simulink model "loopback_delay_estimation"  (R2019b)
settings: Solver=VariableStepAuto  StartTime=0.0  StopTime=18000  RelTol=1e-3
InitFcn:
  | initScript
values from neighbouring files (symbols this model uses):
  bool_ref = (tx_input_ampl_diff<0)    [initScript.m]
  cst = round(scale*cst)    [initScript.m]
  len2 = (len1+d)*L    (= 200)    [initScript.m]
  scale = 30000    [find_corr_threshold.m]    (also in initScript.m = 25000; run_loopback_tests.m = 28000)
  sync_seq_im = int16([cst_im zc_im.' zeros(1, 6000)])    [initScript.m]
  sync_seq_re = int16([cst_re zc_re.' zeros(1, 6000)])    [initScript.m]
  zc_re = round(scale*zc_re/max_val_re)    [initScript.m]
undefined symbols (not defined in the file or in its folder): j
libraries: hdlsllib x11, simulink x6, dsphdlmathfun x2, commsource2 x1, dspsigops x1, commrflib2 x1
settings Model: SimulationMode=accelerator  Creator=spagadar  LastModifiedBy=spagadar
settings OptimizationCC: BlockReduction=off  ConditionallyExecuteInputs=off  DefaultParameterBehavior=Inlined
settings DebuggingCC: AlgebraicLoopMsg=error
settings HardwareCC: ProdBitPerPointer=32  ProdBitPerSizeT=32  ProdBitPerPtrDiffT=32  ProdLargestAtomicFloat=None  ProdIntDivRoundTo=Undefined  ProdEndianess=Unspecified  ProdWordSize=32  ProdHWDeviceType=ASIC/FPGA->ASIC/FPGA  TargetBitPerPointer=64  TargetBitPerSizeT=64  TargetBitPerPtrDiffT=64  TargetLongLongMode=on  TargetIntDivRoundTo=Zero  TargetEndianess=LittleEndian  TargetWordSize=64  TargetHWDeviceType=Custom Processor->MATLAB Host Computer  ProdEqTarget=off

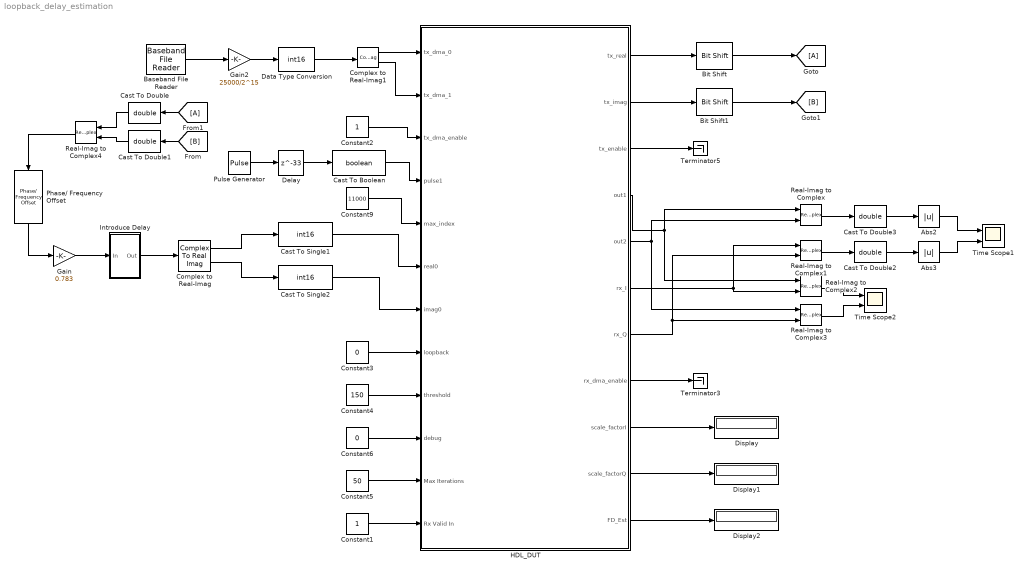
== system loopback_delay_estimation ==
  Abs2 : Abs
  Abs3 : Abs
  Baseband File Reader : commsource2/Baseband File Reader  Filename=zc_out_data_fd.bb  InheritSampleTimeFromFile=on  SampleTime=1  SamplesPerFrame=1  CyclicRepetition=off  FileEndOutputPort=off  SimulateUsing=Code generation
      settings: SourceProductName=Communications Toolbox  SourceProductBaseCode=CM
  Bit Shift : hdlsllib/Logic and Bit Operations/Bit Shift  mode=Shift Right Arithmetic  N=4
      settings: SourceProductName=Simulink
  Bit Shift1 : hdlsllib/Logic and Bit Operations/Bit Shift  mode=Shift Right Arithmetic  N=4
      settings: SourceProductName=Simulink
  Cast To Boolean : DataTypeConversion  OutDataTypeStr=boolean
  Cast To Double{,1..3} (4 alike) : DataTypeConversion  OutDataTypeStr=double
  Cast To Single1 : DataTypeConversion  OutDataTypeStr=int16
  Cast To Single2 : DataTypeConversion  OutDataTypeStr=int16
  Complex to Real-Imag : ComplexToRealImag
  Complex to Real-Imag1 : ComplexToRealImag
  Constant1 : Constant  OutDataTypeStr=boolean  SampleTime=-1
  Constant2 : Constant  OutDataTypeStr=boolean  SampleTime=-1
  Constant3 : Constant  Value=0  OutDataTypeStr=boolean  SampleTime=-1
  Constant4 : Constant  Value=150  OutDataTypeStr=uint16  SampleTime=-1
  Constant5 : Constant  Value=50  OutDataTypeStr=uint16  SampleTime=-1
  Constant6 : Constant  Value=0  OutDataTypeStr=uint16  SampleTime=-1
  Constant9 : Constant  Value=11000  OutDataTypeStr=uint32  SampleTime=-1
  Data Type Conversion : DataTypeConversion  OutDataTypeStr=int16
  Delay : Delay  DelayLength=33
  Display : Display
  Display1 : Display
  Display2 : Display
  Gain : Gain  Gain=0.783
  Gain2 : Gain  Gain=25000/2^15
  HDL_DUT : Subsystem  TreatAsAtomicUnit=on
  Introduce Delay : Subsystem  mask{fd=10, id=146}
      mask prompts: fd "Fractional Delay"; id "Integer Delay"
      mask DialogControl DescTextVar Prompt: Introduce Delay
  Phase/ Frequency Offset : commrflib2/Phase// Frequency Offset  phaseOffset=0  freqPort=off  freqOffset=0
      settings: SourceProductName=Communications Toolbox
  Pulse Generator : DiscretePulseGenerator  Period=16000
  Real-Imag to Complex{,1..4} (5 alike) : RealImagToComplex
  Terminator3 : Terminator
  Terminator5 : Terminator
  Time Scope1 : Scope  NumInputPorts=2
  Time Scope2 : Scope  NumInputPorts=2
  wires:
  [A] -> Cast To Double/1
  [B] -> Cast To Double1/1
  Constant9/1 -> HDL_DUT/5(max_index)
  Complex to Real-Imag/1 -> Cast To Single1/1
  Data Type Conversion/1 -> Complex to Real-Imag1/1
  Constant6/1 -> HDL_DUT/10(debug)
  Complex to Real-Imag1/2 -> HDL_DUT/2(tx_dma_1)
  Cast To Double1/1 -> Real-Imag to Complex4/2
  Cast To Double/1 -> Real-Imag to Complex4/1
  Complex to Real-Imag1/1 -> HDL_DUT/1(tx_dma_0)
  Constant2/1 -> HDL_DUT/3(tx_dma_enable)
  HDL_DUT/1(tx_real) -> Bit Shift/1
  HDL_DUT/2(tx_imag) -> Bit Shift1/1
  Complex to Real-Imag/2 -> Cast To Single2/1
  Constant3/1 -> HDL_DUT/8(loopback)
  Phase/ Frequency Offset/1 -> Gain/1
  Constant4/1 -> HDL_DUT/9(threshold)
  HDL_DUT/8(rx_dma_enable) -> Terminator3/1
  Baseband File Reader/1 -> Gain2/1
  HDL_DUT/3("tx_enable ") -> Terminator5/1
  HDL_DUT/6(rx_I) -> Real-Imag to Complex2/2, Real-Imag to Complex1/1
  HDL_DUT/7(rx_Q) -> Real-Imag to Complex3/2, Real-Imag to Complex1/2
  HDL_DUT/4(out1) -> Real-Imag to Complex2/1, Real-Imag to Complex/1
  HDL_DUT/5(out2) -> Real-Imag to Complex3/1, Real-Imag to Complex/2
  Constant5/1 -> HDL_DUT/11(Max Iterations)
  Abs2/1 -> Time Scope1/1
  Abs3/1 -> Time Scope1/2
  Real-Imag to Complex/1 -> Cast To Double3/1
  Real-Imag to Complex1/1 -> Cast To Double2/1
  Cast To Double2/1 -> Abs3/1
  Cast To Double3/1 -> Abs2/1
  Cast To Single1/1 -> HDL_DUT/6(real0)
  Cast To Single2/1 -> HDL_DUT/7(imag0)
  HDL_DUT/9(scale_factorI) -> Display/1
  Constant1/1 -> HDL_DUT/12(Rx Valid In)
  Real-Imag to Complex2/1 -> Time Scope2/1
  Real-Imag to Complex3/1 -> Time Scope2/2
  HDL_DUT/10(scale_factorQ) -> Display1/1
  Gain2/1 -> Data Type Conversion/1
  HDL_DUT/11(FD_Est) -> Display2/1
  Pulse Generator/1 -> Delay/1
  Cast To Boolean/1 -> HDL_DUT/4(pulse1)
  Delay/1 -> Cast To Boolean/1
  Real-Imag to Complex4/1 -> Phase/ Frequency Offset/1
  Bit Shift/1 -> [A]
  Bit Shift1/1 -> [B]
  Introduce Delay/1(Out) -> Complex to Real-Imag/1
  Gain/1 -> Introduce Delay/1(In)

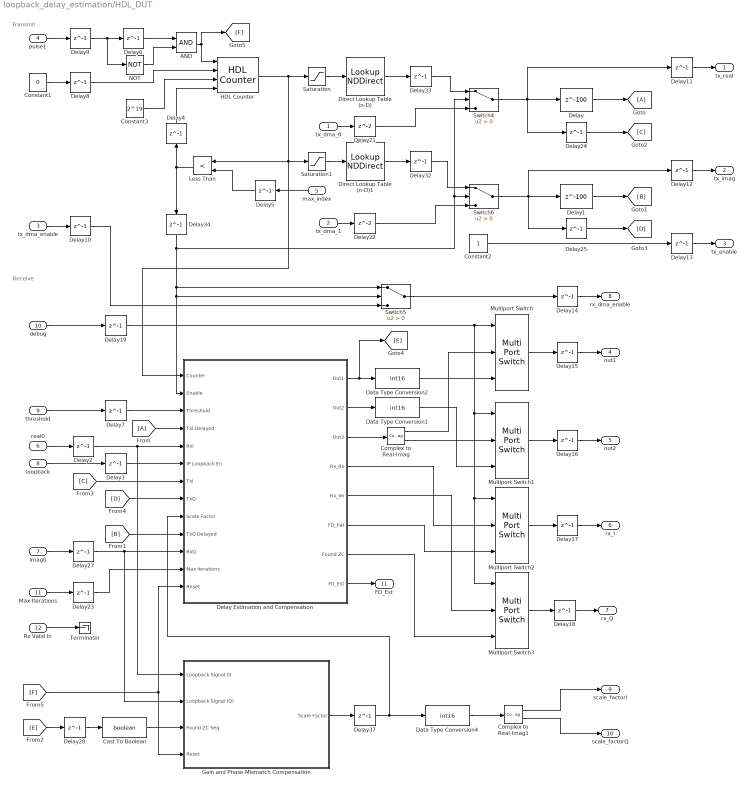
== system loopback_delay_estimation/HDL_DUT ==
  note: Receive
  note: Transmit
  tx_dma_0 : Inport
  tx_dma_1 : Inport  Port=2
  tx_dma_enable : Inport  Port=3
  pulse1 : Inport  Port=4
  max_index : Inport  Port=5  OutDataTypeStr=uint32
  real0 : Inport  Port=6
  imag0 : Inport  Port=7
  loopback : Inport  Port=8  OutDataTypeStr=boolean
  threshold : Inport  Port=9  OutDataTypeStr=uint16
  debug : Inport  Port=10
  Max Iterations : Inport  Port=11  OutDataTypeStr=uint16
  Rx Valid In : Inport  Port=12
  AND : Logic  AllPortsSameDT=off  OutDataTypeStr=boolean
  Cast To Boolean : DataTypeConversion  OutDataTypeStr=boolean
  Complex to Real-Imag : ComplexToRealImag
  Complex to Real-Imag1 : ComplexToRealImag
  Constant1 : Constant  Value=0  OutDataTypeStr=boolean  SampleTime=-1
  Constant2 : Constant  OutDataTypeStr=boolean  SampleTime=-1
  Constant3 : Constant  Value=2^19  OutDataTypeStr=uint32  SampleTime=-1
  Data Type Conversion1 : DataTypeConversion  OutDataTypeStr=int16
  Data Type Conversion2 : DataTypeConversion  OutDataTypeStr=int16
  Data Type Conversion4 : DataTypeConversion  OutDataTypeStr=int16
  Delay : Delay  DelayLength=100  InitialCondition=0  UseCircularBuffer=on
  Delay Estimation and Compensation : Subsystem
  Delay1 : Delay  DelayLength=100  InitialCondition=0  UseCircularBuffer=on
  Delay{2..7,9..19,23..25,27..28,32..34,37} (26 alike) : Delay  DelayLength=1
  Delay21 : Delay
  Delay22 : Delay
  Delay8 : Delay  DelayLength=1  InitialCondition=1
  Direct Lookup Table (n-D) : LookupNDDirect  NumberOfTableDimensions=1  Table=sync_seq_re  DiagnosticForOutOfRangeInput=Error  TableDataTypeStr=int16
  Direct Lookup Table (n-D)1 : LookupNDDirect  NumberOfTableDimensions=1  Table=sync_seq_im  DiagnosticForOutOfRangeInput=Error  TableDataTypeStr=int16
  Gain and Phase Mismatch Compensation : Subsystem
  HDL Counter : hdlsllib/Sources/HDL Counter  CountType=Count limited  CountInit=0  CountStep=1  CountMax=2^20  CountFromType=Initial value  CountFrom=0  CountResetPort=on  CountLoadPort=on  CountEnbPort=on  CountDirPort=off  CountDataType=Unsigned  CountWordLen=32  CountFracLen=0  CountSampTime=1
      settings: SourceProductBaseCode=HD
  Less Than : RelationalOperator  Operator=<  OutDataTypeStr=boolean  RndMeth=Simplest
  Multiport Switch{,1..3} (4 alike) : MultiPortSwitch  DataPortOrder=Zero-based contiguous  Inputs=2  zeroidx=on  OutDataTypeStr=int16
  NOT : Logic  Operator=NOT  IconShape=distinctive  AllPortsSameDT=off  OutDataTypeStr=boolean
  Saturation : Saturate  UpperLimit=999  LowerLimit=0
  Saturation1 : Saturate  UpperLimit=999  LowerLimit=0
  Switch4 : Switch  Criteria=u2 > Threshold
  Switch5 : Switch  Criteria=u2 > Threshold
  Switch6 : Switch  Criteria=u2 > Threshold
  Terminator : Terminator
  tx_real : Outport  VectorParamsAs1DForOutWhenUnconnected=off
  tx_imag : Outport  Port=2  VectorParamsAs1DForOutWhenUnconnected=off
  "tx_enable " : Outport  Port=3  VectorParamsAs1DForOutWhenUnconnected=off
  out1 : Outport  Port=4  OutDataTypeStr=int16  VectorParamsAs1DForOutWhenUnconnected=off
  out2 : Outport  Port=5  VectorParamsAs1DForOutWhenUnconnected=off
  rx_I : Outport  Port=6  VectorParamsAs1DForOutWhenUnconnected=off
  rx_Q : Outport  Port=7  VectorParamsAs1DForOutWhenUnconnected=off
  rx_dma_enable : Outport  Port=8  VectorParamsAs1DForOutWhenUnconnected=off
  scale_factorI : Outport  Port=9  VectorParamsAs1DForOutWhenUnconnected=off
  scale_factorQ : Outport  Port=10  VectorParamsAs1DForOutWhenUnconnected=off
  FD_Est : Outport  Port=11  VectorParamsAs1DForOutWhenUnconnected=off
  wires:
  Direct Lookup Table (n-D)/1 -> Delay33/1
  tx_dma_0/1 -> Delay21/1
  Constant2/1 -> Delay13/1
  loopback/1 -> Delay3/1
  Delay/1 -> [A]
  Delay1/1 -> [B]
  Switch5/1 -> Delay14/1
  tx_dma_enable/1 -> Delay10/1
  Switch4/1 -> Delay11/1, Delay24/1, Delay/1
  Direct Lookup Table (n-D)1/1 -> Delay32/1
  Switch6/1 -> Delay12/1, Delay1/1, Delay25/1
  tx_dma_1/1 -> Delay22/1
  Saturation/1 -> Direct Lookup Table (n-D)/1
  pulse1/1 -> Delay9/1
  Delay6/1 -> AND/1
  NOT/1 -> AND/2
  AND/1 -> [F], HDL Counter/1
  Delay9/1 -> NOT/1, Delay6/1
  Delay10/1 -> Switch5/3
  Delay11/1 -> tx_real/1
  Delay12/1 -> tx_imag/1
  Delay13/1 -> "tx_enable "/1
  Delay14/1 -> rx_dma_enable/1
  Delay15/1 -> out1/1
  Delay16/1 -> out2/1
  Delay17/1 -> rx_I/1
  Delay18/1 -> rx_Q/1
  max_index/1 -> Delay5/1
  Delay21/1 -> Switch4/3
  Delay22/1 -> Switch6/3
  Less Than/1 -> Delay4/1, Delay34/1
  Delay24/1 -> [C]
  Delay25/1 -> [D]
  Delay32/1 -> Switch6/1
  Delay33/1 -> Switch4/1
  Delay4/1 -> HDL Counter/4
  Delay5/1 -> Less Than/2
  [E] -> Delay28/1
  Gain and Phase Mismatch Compensation/1("Scale Factor ") -> Delay37/1
  real0/1 -> Delay2/1
  imag0/1 -> Delay27/1
  Max Iterations/1 -> Delay23/1
  Multiport Switch/1 -> Delay15/1
  Multiport Switch1/1 -> Delay16/1
  Delay28/1 -> Cast To Boolean/1
  Delay Estimation and Compensation/3(Out3) -> Complex to Real-Imag/1
  Delay Estimation and Compensation/2(Out2) -> Data Type Conversion1/1
  Delay Estimation and Compensation/1(Out1) -> [E], Data Type Conversion2/1
  Delay23/1 -> Delay Estimation and Compensation/12(Max Iterations)
  Delay27/1 -> Delay Estimation and Compensation/11(RxQ), Gain and Phase Mismatch Compensation/2(Loopback Signal (Q))
  [B] -> Delay Estimation and Compensation/10(TxQ Delayed)
  Delay37/1 -> Data Type Conversion4/1, Delay Estimation and Compensation/9(Scale Factor)
  [D] -> Delay Estimation and Compensation/8(TxQ)
  [C] -> Delay Estimation and Compensation/7(TxI)
  Delay2/1 -> Delay Estimation and Compensation/5(RxI), Gain and Phase Mismatch Compensation/1(Loopback Signal (I))
  Delay3/1 -> Delay Estimation and Compensation/6(IP Loopback En)
  [A] -> Delay Estimation and Compensation/4(TxI Delayed)
  Delay7/1 -> Delay Estimation and Compensation/3(Threshold)
  Delay34/1 -> Delay Estimation and Compensation/2(Enable), Switch5/2, Switch5/1, Switch4/2, Switch6/2
  Data Type Conversion1/1 -> Multiport Switch1/3
  Data Type Conversion2/1 -> Multiport Switch/3
  HDL Counter/1 -> Saturation1/1, Delay Estimation and Compensation/1(Counter), Less Than/1, Saturation/1
  threshold/1 -> Delay7/1
  Delay19/1 -> Multiport Switch3/1, Multiport Switch2/1, Multiport Switch1/1, Multiport Switch/1
  debug/1 -> Delay19/1
  Multiport Switch3/1 -> Delay18/1
  Multiport Switch2/1 -> Delay17/1
  Delay Estimation and Compensation/4(Rx_Re) -> Multiport Switch2/2
  Delay Estimation and Compensation/5(Rx_Im) -> Multiport Switch3/2
  Cast To Boolean/1 -> Gain and Phase Mismatch Compensation/3(Found ZC Seq)
  Complex to Real-Imag/1 -> Multiport Switch/2
  Complex to Real-Imag/2 -> Multiport Switch1/2
  Rx Valid In/1 -> Terminator/1
  Saturation1/1 -> Direct Lookup Table (n-D)1/1
  Data Type Conversion4/1 -> Complex to Real-Imag1/1
  Complex to Real-Imag1/1 -> scale_factorI/1
  Complex to Real-Imag1/2 -> scale_factorQ/1
  Constant1/1 -> Delay8/1
  Delay8/1 -> HDL Counter/2
  Constant3/1 -> HDL Counter/3
  Delay Estimation and Compensation/8(FD_Est) -> FD_Est/1
  [F] -> Delay Estimation and Compensation/13(Reset), Gain and Phase Mismatch Compensation/4(Reset)
  Delay Estimation and Compensation/6(FD_hat) -> Multiport Switch2/3
  Delay Estimation and Compensation/7(Found ZC) -> Multiport Switch3/3

== system loopback_delay_estimation/Introduce Delay ==
  In : Inport
  Constant8 : Constant  Value=fd/16
  Delay : Delay  DelayLength=id  InitialCondition=0  UseCircularBuffer=on
  Variable Fractional Delay : dspsigops/Variable Fractional Delay  mode=OBSOLETE  modeActive=Linear  L=4  FarrowL=4  R=10  alpha=1  dmax=100  InputProcessing=Columns as channels (frame based)  ic=0  noDFT=off  fallbackFIR=Clip to the minimum value necessary for centered kernel  fallbackFarrow=Clip to the minimum value necessary for centered kernel  roundingMode=Zero  overflowMode=off
      settings: SourceProductName=DSP System Toolbox  SourceProductBaseCode=DS
  Out : Outport  VectorParamsAs1DForOutWhenUnconnected=off
  wires:
  Constant8/1 -> Variable Fractional Delay/2
  In/1 -> Delay/1
  Delay/1 -> Variable Fractional Delay/1
  Variable Fractional Delay/1 -> Out/1

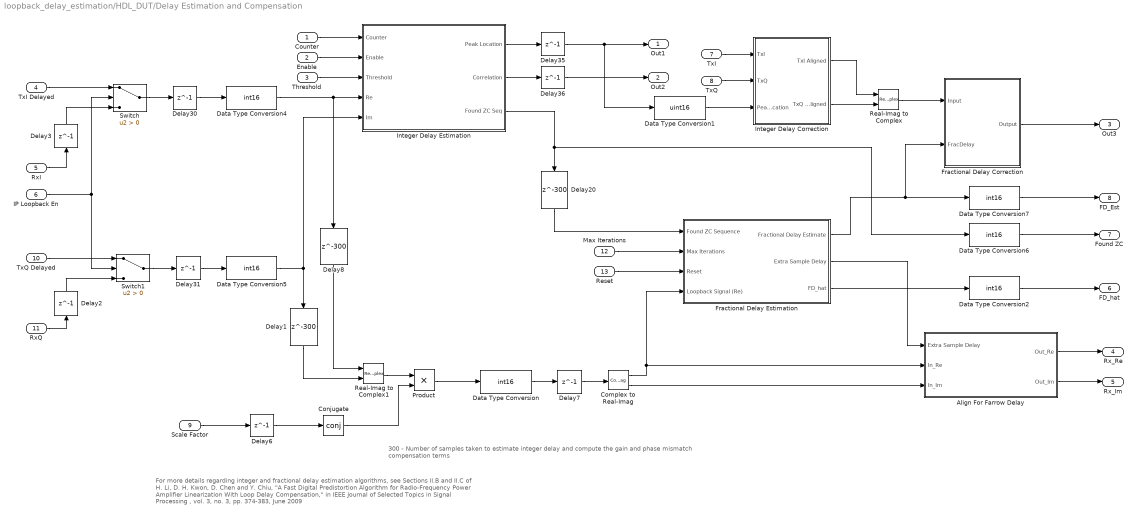
== system loopback_delay_estimation/HDL_DUT/Delay Estimation and Compensation ==
  note: For more details regarding integer and fractional delay estimation algorithms, see Sections II.B and II.C of
      | H. Li, D. H. Kwon, D. Chen and Y. Chiu, "A Fast Digital Predistortion Algorithm for Radio-Frequency Power Amplifier Linearization With Loop Delay Compensation," in IEEE Journal of Selected Topics in Signal Processing , vol. 3, no. 3, pp. 374-383, June 2009
  note: 300 - Number of samples taken to estimate integer delay and compute the gain and phase mismatch compensation terms
  Counter : Inport
  Enable : Inport  Port=2
  Threshold : Inport  Port=3
  TxI Delayed : Inport  Port=4
  RxI : Inport  Port=5
  IP Loopback En : Inport  Port=6
  TxI : Inport  Port=7
  TxQ : Inport  Port=8
  Scale Factor : Inport  Port=9
  TxQ Delayed : Inport  Port=10
  RxQ : Inport  Port=11
  Max Iterations : Inport  Port=12  OutDataTypeStr=uint16
  Reset : Inport  Port=13
  Align For Farrow Delay : Subsystem
  Complex to Real-Imag : ComplexToRealImag
  Conjugate : Math  Operator=conj  RndMeth=Zero  SaturateOnIntegerOverflow=on
  Data Type Conversion{,2,4..7} (6 alike) : DataTypeConversion  OutDataTypeStr=int16
  Data Type Conversion1 : DataTypeConversion  OutDataTypeStr=uint16
  Delay1 : Delay  DelayLength=300  InitialCondition=0  UseCircularBuffer=on
  Delay{2..3,6..7,30..31,35..36} (8 alike) : Delay  DelayLength=1
  Delay20 : Delay  DelayLength=300  InitialCondition=0  UseCircularBuffer=on
  Delay8 : Delay  DelayLength=300  InitialCondition=0  UseCircularBuffer=on
  Fractional Delay Correction : Subsystem  Tag=FilterWizardSubSystem
      settings: ErrorFcn=dspFilterRealizedInBasicElemsAlgLoopErrFcnCallback
  Fractional Delay Estimation : Subsystem
  Integer Delay Correction : Subsystem
  Integer Delay Estimation : Subsystem
  Product : Product
  Real-Imag to Complex : RealImagToComplex
  Real-Imag to Complex1 : RealImagToComplex
  Switch : Switch  Criteria=u2 > Threshold
  Switch1 : Switch  Criteria=u2 > Threshold
  Out1 : Outport
  Out2 : Outport  Port=2
  Out3 : Outport  Port=3
  Rx_Re : Outport  Port=4
  Rx_Im : Outport  Port=5
  FD_hat : Outport  Port=6
  Found ZC : Outport  Port=7
  FD_Est : Outport  Port=8  VectorParamsAs1DForOutWhenUnconnected=off
  wires:
  TxI/1 -> Integer Delay Correction/1(TxI)
  Data Type Conversion4/1 -> Delay8/1, Integer Delay Estimation/4(Re)
  Max Iterations/1 -> Fractional Delay Estimation/2(Max Iterations)
  Delay31/1 -> Data Type Conversion5/1
  Delay30/1 -> Data Type Conversion4/1
  Counter/1 -> Integer Delay Estimation/1(Counter)
  Integer Delay Correction/2(TxQ Aligned) -> Real-Imag to Complex/2
  Integer Delay Correction/1(TxI Aligned) -> Real-Imag to Complex/1
  Fractional Delay Estimation/1(Fractional Delay Estimate) -> Data Type Conversion7/1, Fractional Delay Correction/2(FracDelay)
  Data Type Conversion5/1 -> Integer Delay Estimation/5(Im), Delay1/1
  Fractional Delay Correction/1(Output) -> Out3/1
  Threshold/1 -> Integer Delay Estimation/3(Threshold)
  Delay35/1 -> Data Type Conversion1/1, Out1/1
  Switch1/1 -> Delay31/1
  Integer Delay Estimation/2(Correlation) -> Delay36/1
  Enable/1 -> Integer Delay Estimation/2(Enable)
  Delay36/1 -> Out2/1
  Real-Imag to Complex/1 -> Fractional Delay Correction/1(Input)
  TxQ Delayed/1 -> Switch1/1
  RxI/1 -> Delay3/1
  Integer Delay Estimation/1(Peak Location) -> Delay35/1
  TxI Delayed/1 -> Switch/1
  IP Loopback En/1 -> Switch1/2, Switch/2
  RxQ/1 -> Delay2/1
  TxQ/1 -> Integer Delay Correction/2(TxQ)
  Switch/1 -> Delay30/1
  Delay20/1 -> Fractional Delay Estimation/1(Found ZC Sequence)
  Delay3/1 -> Switch/3
  Delay2/1 -> Switch1/3
  Delay8/1 -> Real-Imag to Complex1/1
  Scale Factor/1 -> Delay6/1
  Delay1/1 -> Real-Imag to Complex1/2
  Data Type Conversion1/1 -> Integer Delay Correction/3(Peak Location)
  Complex to Real-Imag/1 -> Align For Farrow Delay/2(In_Re), Fractional Delay Estimation/4(Loopback Signal (Re))
  Data Type Conversion/1 -> Delay7/1
  Delay6/1 -> Conjugate/1
  Product/1 -> Data Type Conversion/1
  Delay7/1 -> Complex to Real-Imag/1
  Data Type Conversion2/1 -> FD_hat/1
  Conjugate/1 -> Product/2
  Real-Imag to Complex1/1 -> Product/1
  Data Type Conversion6/1 -> Found ZC/1
  Integer Delay Estimation/3(Found ZC Seq) -> Data Type Conversion6/1, Delay20/1
  Fractional Delay Estimation/3(FD_hat) -> Data Type Conversion2/1
  Fractional Delay Estimation/2(Extra Sample Delay) -> Align For Farrow Delay/1(Extra Sample Delay)
  Complex to Real-Imag/2 -> Align For Farrow Delay/3(In_Im)
  Align For Farrow Delay/1(Out_Re) -> Rx_Re/1
  Align For Farrow Delay/2(Out_Im) -> Rx_Im/1
  Reset/1 -> Fractional Delay Estimation/3(Reset)
  Data Type Conversion7/1 -> FD_Est/1

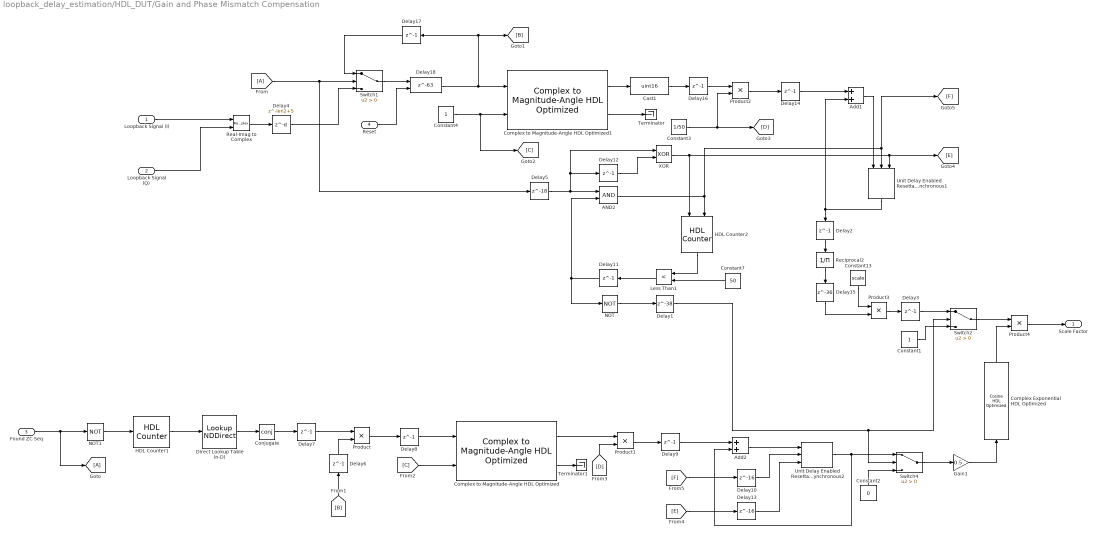
== system loopback_delay_estimation/HDL_DUT/Gain and Phase Mismatch Compensation ==
  Loopback Signal (I) : Inport
  Loopback Signal (Q) : Inport  Port=2
  Found ZC Seq : Inport  Port=3
  Reset : Inport  Port=4
  AND2 : Logic  AllPortsSameDT=off  OutDataTypeStr=boolean
  Add1 : Sum  OutDataTypeStr=uint32
  Add2 : Sum  OutDataTypeStr=fixdt(0,16,13)
  Cast1 : DataTypeConversion  OutDataTypeStr=uint16
  Complex Exponential HDL Optimized : hdlsllib/Lookup Tables/Cosine HDL Optimized  OutputFormula=exp(j*2*pi*u)  NumDataPoints=512  TableDataTypeStr=fixdt(0,16,15)  SimulateLUTROMDelay=off
      settings: SourceProductName=Simulink  SourceProductBaseCode=SL
  Complex to Magnitude-Angle HDL Optimized : dsphdlmathfun/Complex to Magnitude-Angle HDL Optimized  NumIterationsSource=Auto  NumIterations=10  OutputFormat=Angle  AngleFormat=Normalized  ScaleOutput=off  SimulateUsing=Code generation
      settings: SourceProductName=DSP System Toolbox  SourceProductBaseCode=DS
  Complex to Magnitude-Angle HDL Optimized1 : dsphdlmathfun/Complex to Magnitude-Angle HDL Optimized  NumIterationsSource=Auto  NumIterations=10  OutputFormat=Magnitude  AngleFormat=Radians  ScaleOutput=on  SimulateUsing=Code generation
      settings: SourceProductName=DSP System Toolbox  SourceProductBaseCode=DS
  Conjugate : Math  Operator=conj  RndMeth=Zero  SaturateOnIntegerOverflow=on
  Constant1 : Constant  OutDataTypeStr=uint16  SampleTime=-1
  Constant13 : Constant  Value=scale  OutDataTypeStr=uint16  SampleTime=-1
  Constant2 : Constant  Value=0  OutDataTypeStr=uint16  SampleTime=-1
  Constant3 : Constant  Value=1/50  OutDataTypeStr=fixdt(1,16,16)  SampleTime=-1
  Constant4 : Constant  OutDataTypeStr=boolean  SampleTime=-1
  Constant7 : Constant  Value=50  OutDataTypeStr=uint8  SampleTime=-1
  Delay1 : Delay  DelayLength=38
  Delay10 : Delay  DelayLength=16
  Delay{2..3,6..9,11..12,14,16..17} (11 alike) : Delay  DelayLength=1
  Delay13 : Delay  DelayLength=16
  Delay15 : Delay  DelayLength=36
  Delay18 : Delay  DelayLength=63  ExternalReset=Level
      settings: InputPortMap=u0,r5
  Delay4 : Delay  DelayLength=len2+5
  Delay5 : Delay  DelayLength=18
  Direct Lookup Table (n-D) : LookupNDDirect  NumberOfTableDimensions=1  Table=cst  DiagnosticForOutOfRangeInput=Error  TableDataTypeStr=int16
  Gain1 : Gain  Gain=0.5
  HDL Counter1 : hdlsllib/Sources/HDL Counter  CountType=Count limited  CountInit=0  CountStep=1  CountMax=63  CountFromType=Initial value  CountFrom=0  CountResetPort=on  CountLoadPort=off  CountEnbPort=off  CountDirPort=off  CountDataType=Unsigned  CountWordLen=8  CountFracLen=0  CountSampTime=1
      settings: SourceProductName=Simulink
  HDL Counter2 : hdlsllib/Sources/HDL Counter  CountType=Count limited  CountInit=0  CountStep=1  CountMax=60  CountFromType=Initial value  CountFrom=0  CountResetPort=on  CountLoadPort=off  CountEnbPort=on  CountDirPort=off  CountDataType=Unsigned  CountWordLen=8  CountFracLen=0  CountSampTime=1
      settings: SourceProductName=Simulink
  Less Than1 : RelationalOperator  Operator=<  OutDataTypeStr=boolean  RndMeth=Simplest
  NOT : Logic  Operator=NOT  AllPortsSameDT=off  OutDataTypeStr=boolean
  NOT1 : Logic  Operator=NOT  AllPortsSameDT=off  OutDataTypeStr=boolean
  Product{,1,3..4} (4 alike) : Product
  Product2 : Product  OutDataTypeStr=fixdt(0,16,7)
  Real-Imag to Complex : RealImagToComplex
  Reciprocal2 : Product  Inputs=/  SaturateOnIntegerOverflow=on  RndMeth=Zero
  Switch1 : Switch  Criteria=u2 > Threshold
  Switch2 : Switch  Criteria=u2 > Threshold  OutDataTypeStr=fixdt(0,16,7)
  Switch4 : Switch  Criteria=u2 > Threshold  OutDataTypeStr=fixdt(0,16,13)
  Terminator : Terminator
  Terminator1 : Terminator
  Unit Delay Enabled Resettable Synchronous1 : hdlsllib/Discrete/Unit Delay Enabled Resettable Synchronous  InitialCondition=0  SampleTime=-1
      settings: SourceProductName=Simulink  SourceProductBaseCode=SL
  Unit Delay Enabled Resettable Synchronous2 : hdlsllib/Discrete/Unit Delay Enabled Resettable Synchronous  InitialCondition=0  SampleTime=-1
      settings: SourceProductName=Simulink  SourceProductBaseCode=SL
  XOR : Logic  Operator=XOR  AllPortsSameDT=off  OutDataTypeStr=boolean
  "Scale Factor " : Outport
  wires:
  Loopback Signal (I)/1 -> Real-Imag to Complex/1
  Loopback Signal (Q)/1 -> Real-Imag to Complex/2
  Real-Imag to Complex/1 -> Delay4/1
  Reciprocal2/1 -> Delay15/1
  Less Than1/1 -> Delay11/1
  Unit Delay Enabled Resettable Synchronous1/1 -> Add1/2, Delay2/1
  HDL Counter2/1 -> Less Than1/1
  Constant7/1 -> Less Than1/2
  Constant3/1 -> [D], Product2/2
  Delay12/1 -> XOR/2
  Delay15/1 -> Product3/2
  Product2/1 -> Delay14/1
  Constant4/1 -> [C], Complex to Magnitude-Angle HDL Optimized1/2
  Switch1/1 -> Delay18/1
  Delay16/1 -> Product2/1
  Constant13/1 -> Product3/1
  XOR/1 -> HDL Counter2/1, [E], Unit Delay Enabled Resettable Synchronous1/3
  Cast1/1 -> Delay16/1
  Complex to Magnitude-Angle HDL Optimized1/1 -> Cast1/1
  Delay14/1 -> Add1/1
  Delay11/1 -> AND2/2, NOT/1
  Add1/1 -> Unit Delay Enabled Resettable Synchronous1/1
  Complex to Magnitude-Angle HDL Optimized1/2 -> Terminator/1
  Switch2/1 -> Product4/1
  Product3/1 -> Delay3/1
  Constant1/1 -> Switch2/3
  Delay1/1 -> Switch4/2, Switch2/2
  Delay2/1 -> Reciprocal2/1
  Delay3/1 -> Switch2/1
  Delay4/1 -> Switch1/3
  Delay5/1 -> AND2/1, XOR/1, Delay12/1
  NOT/1 -> Delay1/1
  Found ZC Seq/1 -> NOT1/1, [A]
  NOT1/1 -> HDL Counter1/1
  HDL Counter1/1 -> Direct Lookup Table (n-D)/1
  Conjugate/1 -> Delay7/1
  Product/1 -> Delay8/1
  Complex to Magnitude-Angle HDL Optimized/1 -> Product1/1
  Delay18/1 -> [B], Delay17/1, Complex to Magnitude-Angle HDL Optimized1/1
  Direct Lookup Table (n-D)/1 -> Conjugate/1
  Delay7/1 -> Product/1
  Delay6/1 -> Product/2
  Delay8/1 -> Complex to Magnitude-Angle HDL Optimized/1
  Product1/1 -> Delay9/1
  Delay9/1 -> Add2/1
  Add2/1 -> Unit Delay Enabled Resettable Synchronous2/1
  AND2/1 -> HDL Counter2/2, [F], Unit Delay Enabled Resettable Synchronous1/2
  Delay10/1 -> Unit Delay Enabled Resettable Synchronous2/2
  Delay13/1 -> Unit Delay Enabled Resettable Synchronous2/3
  Unit Delay Enabled Resettable Synchronous2/1 -> Add2/2, Switch4/1
  Constant2/1 -> Switch4/3
  Product4/1 -> "Scale Factor "/1
  Complex to Magnitude-Angle HDL Optimized/2 -> Terminator1/1
  [A] -> Delay5/1, Switch1/2
  [B] -> Delay6/1
  [C] -> Complex to Magnitude-Angle HDL Optimized/2
  [D] -> Product1/2
  [E] -> Delay13/1
  [F] -> Delay10/1
  Switch4/1 -> Gain1/1
  Complex Exponential HDL Optimized/1 -> Product4/2
  Gain1/1 -> Complex Exponential HDL Optimized/1
  Delay17/1 -> Switch1/1
  Reset/1 -> Delay18/2

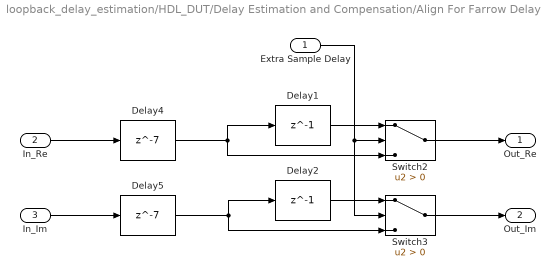
== system loopback_delay_estimation/HDL_DUT/Delay Estimation and Compensation/Align For Farrow Delay ==
  Extra Sample Delay : Inport
  In_Re : Inport  Port=2
  In_Im : Inport  Port=3
  Delay1 : Delay  DelayLength=1  InitialCondition=0  UseCircularBuffer=on
  Delay2 : Delay  DelayLength=1  InitialCondition=0  UseCircularBuffer=on
  Delay4 : Delay  DelayLength=7  InitialCondition=0  UseCircularBuffer=on
  Delay5 : Delay  DelayLength=7  InitialCondition=0  UseCircularBuffer=on
  Switch2 : Switch  Criteria=u2 > Threshold
  Switch3 : Switch  Criteria=u2 > Threshold
  Out_Re : Outport
  Out_Im : Outport  Port=2
  wires:
  Delay5/1 -> Delay2/1, Switch3/3
  Delay4/1 -> Delay1/1, Switch2/3
  Switch3/1 -> Out_Im/1
  Extra Sample Delay/1 -> Switch3/2, Switch2/2
  In_Re/1 -> Delay4/1
  Switch2/1 -> Out_Re/1
  In_Im/1 -> Delay5/1
  Delay1/1 -> Switch2/1
  Delay2/1 -> Switch3/1

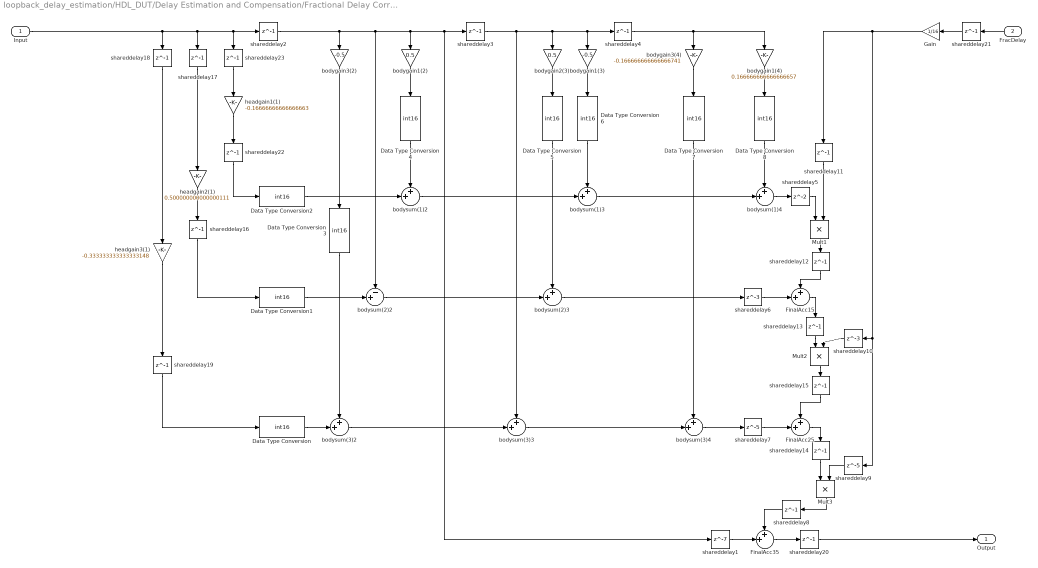
== system loopback_delay_estimation/HDL_DUT/Delay Estimation and Compensation/Fractional Delay Correction ==
  Input : Inport
  FracDelay : Inport  Port=2
  Data Type Conversion{,1..8} (9 alike) : DataTypeConversion  OutDataTypeStr=int16
  FinalAcc15 : Sum  Inputs=++|  RndMeth=Nearest  SaturateOnIntegerOverflow=on
  FinalAcc25 : Sum  Inputs=++|  RndMeth=Nearest  SaturateOnIntegerOverflow=on
  FinalAcc35 : Sum  Inputs=++|  RndMeth=Nearest  SaturateOnIntegerOverflow=on  OutDataTypeStr=Inherit: Same as first input
  Gain : Gain  Gain=1/16
  Mult1 : Product  RndMeth=Nearest  SaturateOnIntegerOverflow=on  OutDataTypeStr=Inherit: Same as first input
  Mult2 : Product  RndMeth=Nearest  SaturateOnIntegerOverflow=on  OutDataTypeStr=Inherit: Same as first input
  Mult3 : Product  RndMeth=Nearest  SaturateOnIntegerOverflow=on  OutDataTypeStr=Inherit: Same as first input
  bodygain1(2) : Gain  Gain=0.5  SaturateOnIntegerOverflow=on
  bodygain1(3) : Gain  Gain=-0.5  SaturateOnIntegerOverflow=on
  bodygain1(4) : Gain  Gain=0.166666666666666657  SaturateOnIntegerOverflow=on
  bodygain2(3) : Gain  Gain=0.5  SaturateOnIntegerOverflow=on
  bodygain3(2) : Gain  Gain=-0.5  SaturateOnIntegerOverflow=on
  bodygain3(4) : Gain  Gain=-0.166666666666666741  SaturateOnIntegerOverflow=on
  bodysum(1)2 : Sum  Inputs=++|  RndMeth=Nearest  SaturateOnIntegerOverflow=on
  bodysum(1)3 : Sum  Inputs=++|  RndMeth=Nearest  SaturateOnIntegerOverflow=on
  bodysum(1)4 : Sum  Inputs=++|  RndMeth=Nearest  SaturateOnIntegerOverflow=on
  bodysum(2)2 : Sum  Inputs=-+|  RndMeth=Nearest  SaturateOnIntegerOverflow=on
  bodysum(2)3 : Sum  Inputs=++|  RndMeth=Nearest  SaturateOnIntegerOverflow=on
  bodysum(3)2 : Sum  Inputs=++|  RndMeth=Nearest  SaturateOnIntegerOverflow=on
  bodysum(3)3 : Sum  Inputs=++|  RndMeth=Nearest  SaturateOnIntegerOverflow=on
  bodysum(3)4 : Sum  Inputs=++|  RndMeth=Nearest  SaturateOnIntegerOverflow=on
  headgain1(1) : Gain  Gain=-0.16666666666666663  SaturateOnIntegerOverflow=on
  headgain2(1) : Gain  Gain=0.500000000000000111  SaturateOnIntegerOverflow=on
  headgain3(1) : Gain  Gain=-0.333333333333333148  SaturateOnIntegerOverflow=on
  shareddelay1 : Delay  DelayLength=7  InitialCondition=0  InputProcessing=Columns as channels (frame based)
  shareddelay10 : Delay  DelayLength=3  InitialCondition=0  InputProcessing=Columns as channels (frame based)
  shareddelay{2..4,8,11..23} (17 alike) : Delay  DelayLength=1  InitialCondition=0  InputProcessing=Columns as channels (frame based)
  shareddelay5 : Delay  InitialCondition=0  InputProcessing=Columns as channels (frame based)
  shareddelay6 : Delay  DelayLength=3  InitialCondition=0  InputProcessing=Columns as channels (frame based)
  shareddelay7 : Delay  DelayLength=5  InitialCondition=0  InputProcessing=Columns as channels (frame based)
  shareddelay9 : Delay  DelayLength=5  InitialCondition=0  InputProcessing=Columns as channels (frame based)
  Output : Outport  VectorParamsAs1DForOutWhenUnconnected=off
  wires:
  bodysum(1)2/1 -> bodysum(1)3/2
  bodysum(2)2/1 -> bodysum(2)3/2
  bodysum(3)2/1 -> bodysum(3)3/2
  bodysum(1)3/1 -> bodysum(1)4/2
  bodysum(2)3/1 -> shareddelay6/1
  bodysum(3)3/1 -> bodysum(3)4/2
  bodygain3(4)/1 -> Data Type Conversion7/1
  bodysum(1)4/1 -> shareddelay5/1
  bodysum(3)4/1 -> shareddelay7/1
  shareddelay4/1 -> bodygain1(4)/1, bodygain3(4)/1
  FracDelay/1 -> shareddelay21/1
  Mult1/1 -> shareddelay12/1
  FinalAcc15/1 -> shareddelay13/1
  Mult2/1 -> shareddelay15/1
  FinalAcc25/1 -> shareddelay14/1
  Mult3/1 -> shareddelay8/1
  shareddelay20/1 -> Output/1
  FinalAcc35/1 -> shareddelay20/1
  Gain/1 -> shareddelay9/1, shareddelay10/1, shareddelay11/1
  Input/1 -> shareddelay23/1, shareddelay2/1, shareddelay17/1, shareddelay18/1
  shareddelay1/1 -> FinalAcc35/2
  shareddelay7/1 -> FinalAcc25/2
  shareddelay6/1 -> FinalAcc15/2
  shareddelay5/1 -> Mult1/1
  headgain3(1)/1 -> shareddelay19/1
  bodygain3(2)/1 -> Data Type Conversion3/1
  shareddelay3/1 -> bodysum(3)3/1, bodygain1(3)/1, shareddelay4/1, bodygain2(3)/1
  Data Type Conversion7/1 -> bodysum(3)4/1
  headgain2(1)/1 -> shareddelay16/1
  shareddelay2/1 -> shareddelay3/1, shareddelay1/1, bodygain1(2)/1, bodysum(2)2/1, bodygain3(2)/1
  bodygain2(3)/1 -> Data Type Conversion5/1
  headgain1(1)/1 -> shareddelay22/1
  bodygain1(2)/1 -> Data Type Conversion4/1
  bodygain1(4)/1 -> Data Type Conversion8/1
  bodygain1(3)/1 -> Data Type Conversion6/1
  Data Type Conversion/1 -> bodysum(3)2/2
  Data Type Conversion1/1 -> bodysum(2)2/2
  Data Type Conversion2/1 -> bodysum(1)2/2
  Data Type Conversion3/1 -> bodysum(3)2/1
  Data Type Conversion4/1 -> bodysum(1)2/1
  Data Type Conversion5/1 -> bodysum(2)3/1
  Data Type Conversion6/1 -> bodysum(1)3/1
  Data Type Conversion8/1 -> bodysum(1)4/1
  shareddelay21/1 -> Gain/1
  shareddelay8/1 -> FinalAcc35/1
  shareddelay9/1 -> Mult3/2
  shareddelay10/1 -> Mult2/2
  shareddelay11/1 -> Mult1/2
  shareddelay12/1 -> FinalAcc15/1
  shareddelay13/1 -> Mult2/1
  shareddelay14/1 -> Mult3/1
  shareddelay15/1 -> FinalAcc25/1
  shareddelay19/1 -> Data Type Conversion/1
  shareddelay18/1 -> headgain3(1)/1
  shareddelay17/1 -> headgain2(1)/1
  shareddelay16/1 -> Data Type Conversion1/1
  shareddelay23/1 -> headgain1(1)/1
  shareddelay22/1 -> Data Type Conversion2/1

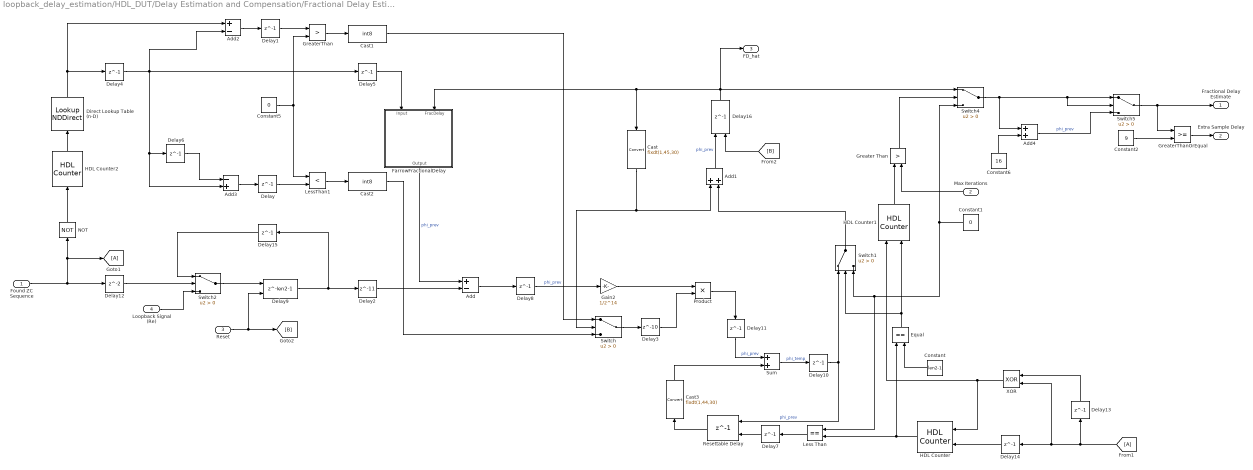
== system loopback_delay_estimation/HDL_DUT/Delay Estimation and Compensation/Fractional Delay Estimation ==
  Found ZC Sequence : Inport
  Max Iterations : Inport  Port=2
  Reset : Inport  Port=3
  Loopback Signal (Re) : Inport  Port=4
  Add : Sum  Inputs=+-
  Add1 : Sum
  Add2 : Sum  Inputs=+-
  Add3 : Sum  Inputs=-+
  Add4 : Sum  OutDataTypeStr=fixdt(0,46,30)
  Cast : DataTypeConversion  OutDataTypeStr=fixdt(1,45,30)
  Cast1 : DataTypeConversion  OutDataTypeStr=int8
  Cast2 : DataTypeConversion  OutDataTypeStr=int8
  Cast3 : DataTypeConversion  OutDataTypeStr=fixdt(1,44,30)
  Constant : Constant  Value=len2-1  OutDataTypeStr=uint16  SampleTime=-1
  Constant1 : Constant  Value=0  OutDataTypeStr=Inherit: Inherit via back propagation  SampleTime=-1
  Constant2 : Constant  Value=9  OutDataTypeStr=uint8  SampleTime=-1
  Constant5 : Constant  Value=0  OutDataTypeStr=boolean  SampleTime=-1
  Constant6 : Constant  Value=16  OutDataTypeStr=fixdt(1,46,30)  SampleTime=-1
  Delay{,1,4..8,10..11,13..15} (12 alike) : Delay  DelayLength=1
  Delay12 : Delay
  Delay16 : Delay  DelayLength=1  ExternalReset=Level  UseCircularBuffer=on
      settings: InputPortMap=u0,r5
  Delay2 : Delay  DelayLength=11
  Delay3 : Delay  DelayLength=10
  Delay9 : Delay  DelayLength=len2-1  ExternalReset=Level  UseCircularBuffer=on
      settings: InputPortMap=u0,r5
  Direct Lookup Table (n-D) : LookupNDDirect  NumberOfTableDimensions=1  Table=zc_re  DiagnosticForOutOfRangeInput=Error  TableDataTypeStr=int16
  Equal : RelationalOperator  Operator===  OutDataTypeStr=boolean  RndMeth=Simplest
  FarrowFractionalDelay : Subsystem  Tag=FilterWizardSubSystem
      settings: ErrorFcn=dspFilterRealizedInBasicElemsAlgLoopErrFcnCallback
  Gain2 : Gain  Gain=1/2^14
  Greater Than : RelationalOperator  Operator=>  OutDataTypeStr=boolean  RndMeth=Simplest
  GreaterThan : RelationalOperator  Operator=>  OutDataTypeStr=boolean  RndMeth=Simplest
  GreaterThanOrEqual : RelationalOperator  OutDataTypeStr=boolean  RndMeth=Simplest
  HDL Counter : hdlsllib/Sources/HDL Counter  CountType=Count limited  CountInit=0  CountStep=1  CountMax=len2-1  CountFromType=Initial value  CountFrom=0  CountResetPort=on  CountLoadPort=off  CountEnbPort=on  CountDirPort=off  CountDataType=Unsigned  CountWordLen=16  CountFracLen=0  CountSampTime=1
      settings: SourceProductName=Simulink
  HDL Counter1 : hdlsllib/Sources/HDL Counter  CountType=Count limited  CountInit=0  CountStep=1  CountMax=2^16-1  CountFromType=Initial value  CountFrom=0  CountResetPort=on  CountLoadPort=off  CountEnbPort=on  CountDirPort=off  CountDataType=Unsigned  CountWordLen=16  CountFracLen=0  CountSampTime=1
      settings: SourceProductName=Simulink
  HDL Counter2 : hdlsllib/Sources/HDL Counter  CountType=Count limited  CountInit=1  CountStep=1  CountMax=len2  CountFromType=Initial value  CountFrom=1  CountResetPort=on  CountLoadPort=off  CountEnbPort=off  CountDirPort=off  CountDataType=Unsigned  CountWordLen=16  CountFracLen=0  CountSampTime=1
      settings: SourceProductName=Simulink
  Less Than : RelationalOperator  Operator===  OutDataTypeStr=boolean  RndMeth=Simplest
  LessThan1 : RelationalOperator  Operator=<  OutDataTypeStr=boolean  RndMeth=Simplest
  NOT : Logic  Operator=NOT  AllPortsSameDT=off  OutDataTypeStr=boolean
  Product : Product
  Resettable Delay : Delay  DelayLength=1  ExternalReset=Level
      settings: InputPortMap=u0,r5
  Sum : Sum
  Switch{,1..2,4..5} (5 alike) : Switch  Criteria=u2 > Threshold
  XOR : Logic  Operator=XOR  AllPortsSameDT=off  OutDataTypeStr=boolean
  Fractional Delay Estimate : Outport
  Extra Sample Delay : Outport  Port=2
  FD_hat : Outport  Port=3
  wires:
  Add3/1 -> Delay/1
  GreaterThan/1 -> Cast1/1
  Cast1/1 -> Switch/1
  Constant1/1 -> Switch1/3, Less Than/1, Switch4/3
  Cast2/1 -> Switch/3
  Constant5/1 -> LessThan1/1, GreaterThan/2
  LessThan1/1 -> Cast2/1
  Gain2/1 -> Product/1
  Sum/1 -> Delay10/1  "phi_temp"
  HDL Counter/1 -> Equal/1, Less Than/2
  HDL Counter1/1 -> Greater Than/1
  Resettable Delay/1 -> Cast3/1
  Less Than/1 -> Delay7/1
  Add2/1 -> Delay1/1
  HDL Counter2/1 -> Direct Lookup Table (n-D)/1
  Switch1/1 -> Add1/2
  Add/1 -> Delay8/1
  Switch/1 -> Delay3/1
  Delay2/1 -> Add/2
  Delay4/1 -> Add2/2, Add3/2, Delay6/1, Delay5/1
  Equal/1 -> HDL Counter1/2, Switch1/2
  Direct Lookup Table (n-D)/1 -> Delay4/1, Add2/1
  Greater Than/1 -> Switch4/2
  Max Iterations/1 -> Greater Than/2
  Product/1 -> Delay11/1
  Delay7/1 -> Resettable Delay/2
  Delay3/1 -> Product/2
  Add1/1 -> Delay16/1  "phi_prev"
  Delay8/1 -> Gain2/1  "phi_prev"
  Delay1/1 -> GreaterThan/1
  Delay/1 -> LessThan1/2
  Delay11/1 -> Sum/1  "phi_prev"
  Delay10/1 -> Resettable Delay/1, Switch1/1  "phi_prev"
  Found ZC Sequence/1 -> NOT/1, [A], Delay12/1
  XOR/1 -> HDL Counter/1, HDL Counter1/1
  Delay14/1 -> HDL Counter/2
  Delay13/1 -> XOR/1
  Cast/1 -> Switch/2, Add1/1
  Delay5/1 -> FarrowFractionalDelay/1(Input)
  Add4/1 -> Switch5/3  "phi_prev"
  Constant6/1 -> Add4/2
  Switch4/1 -> Add4/1, Switch5/2, Switch5/1
  GreaterThanOrEqual/1 -> Extra Sample Delay/1
  NOT/1 -> HDL Counter2/1
  Switch5/1 -> GreaterThanOrEqual/1, Fractional Delay Estimate/1
  Delay9/1 -> Delay15/1, Delay2/1
  Loopback Signal (Re)/1 -> Switch2/3
  Switch2/1 -> Delay9/1
  Delay15/1 -> Switch2/1
  Delay12/1 -> Switch2/2
  FarrowFractionalDelay/1(Output) -> Add/1  "phi_prev"
  [A] -> XOR/2, Delay14/1, Delay13/1
  Constant/1 -> Equal/2
  Delay16/1 -> Cast/1, FarrowFractionalDelay/2(FracDelay), FD_hat/1, Switch4/1
  Cast3/1 -> Sum/2
  Delay6/1 -> Add3/1
  Reset/1 -> [B], Delay9/2
  [B] -> Delay16/2
  Constant2/1 -> GreaterThanOrEqual/2

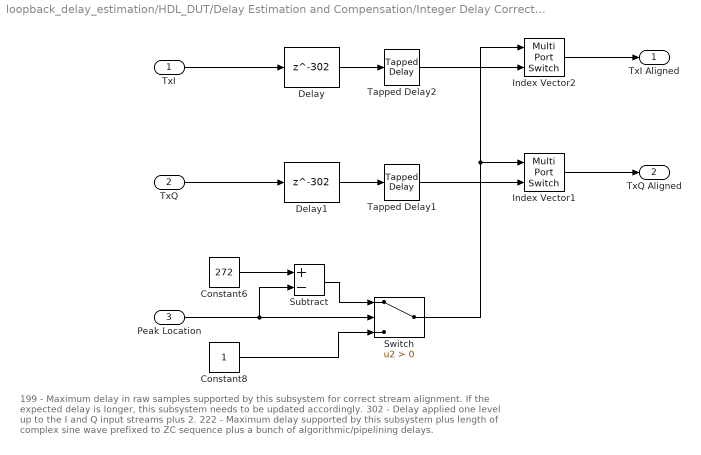
== system loopback_delay_estimation/HDL_DUT/Delay Estimation and Compensation/Integer Delay Correction ==
  note: 199 - Maximum delay in raw samples supported by this subsystem for correct stream alignment. If the expected delay is longer, this subsystem needs to be updated accordingly.
      | 302 - Delay applied one level up to the I and Q input streams plus 2.
      | 222 - Maximum delay supported by this subsystem plus length of complex sine wave prefixed to ZC sequence plus a bunch of algorithmic/pipelining delays.
  TxI : Inport
  TxQ : Inport  Port=2
  Peak Location : Inport  Port=3
  Constant6 : Constant  Value=272  OutDataTypeStr=uint16  SampleTime=-1
  Constant8 : Constant  OutDataTypeStr=uint16  SampleTime=-1
  Delay : Delay  DelayLength=302  InitialCondition=0  UseCircularBuffer=on
  Delay1 : Delay  DelayLength=302  InitialCondition=0  UseCircularBuffer=on
  Index Vector1 : MultiPortSwitch  Inputs=1
  Index Vector2 : MultiPortSwitch  Inputs=1
  Subtract : Sum  Inputs=+-
  Switch : Switch  Criteria=u2 > Threshold
  Tapped Delay1 : simulink/Discrete/Tapped Delay  vinit=0.0  samptime=-1  NumDelays=200  DelayOrder=Oldest  includeCurrent=off
  Tapped Delay2 : simulink/Discrete/Tapped Delay  vinit=0.0  samptime=-1  NumDelays=200  DelayOrder=Oldest  includeCurrent=off
  TxI Aligned : Outport  VectorParamsAs1DForOutWhenUnconnected=off
  TxQ Aligned : Outport  Port=2  VectorParamsAs1DForOutWhenUnconnected=off
  wires:
  Delay/1 -> Tapped Delay2/1
  Index Vector2/1 -> TxI Aligned/1
  TxI/1 -> Delay/1
  TxQ/1 -> Delay1/1
  Delay1/1 -> Tapped Delay1/1
  Index Vector1/1 -> TxQ Aligned/1
  Peak Location/1 -> Switch/2, Subtract/2
  Subtract/1 -> Switch/1
  Constant8/1 -> Switch/3
  Switch/1 -> Index Vector1/1, Index Vector2/1
  Constant6/1 -> Subtract/1
  Tapped Delay1/1 -> Index Vector1/2
  Tapped Delay2/1 -> Index Vector2/2

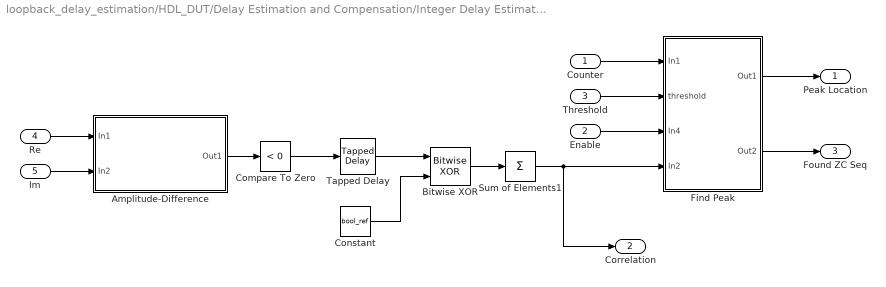
== system loopback_delay_estimation/HDL_DUT/Delay Estimation and Compensation/Integer Delay Estimation ==
  Counter : Inport
  Enable : Inport  Port=2
  Threshold : Inport  Port=3
  Re : Inport  Port=4
  Im : Inport  Port=5
  Amplitude-Difference : Subsystem
  Bitwise XOR : simulink/Logic and Bit Operations/Bitwise Operator  logicop=XOR  UseBitMask=off  NumInputPorts=2  BitMask=bin2dec('11011')  BitMaskRealWorld=Stored Integer
  Compare To Zero : simulink/Logic and Bit Operations/Compare To Zero  relop=<  OutDataTypeStr=boolean
  Constant : Constant  Value=bool_ref  OutDataTypeStr=boolean  SampleTime=1
  Find Peak : Subsystem
  Sum of Elements1 : Sum  Inputs=+  AccumDataTypeStr=uint8
  Tapped Delay : simulink/Discrete/Tapped Delay  vinit=0.0  samptime=-1  NumDelays=len2-1  DelayOrder=Oldest  includeCurrent=off
  Peak Location : Outport  VectorParamsAs1DForOutWhenUnconnected=off
  Correlation : Outport  Port=2  VectorParamsAs1DForOutWhenUnconnected=off
  Found ZC Seq : Outport  Port=3  VectorParamsAs1DForOutWhenUnconnected=off
  wires:
  Amplitude-Difference/1(Out1) -> Compare To Zero/1
  Re/1 -> Amplitude-Difference/1(In1)
  Im/1 -> Amplitude-Difference/2(In2)
  Bitwise XOR/1 -> Sum of Elements1/1
  Constant/1 -> Bitwise XOR/2
  Tapped Delay/1 -> Bitwise XOR/1
  Compare To Zero/1 -> Tapped Delay/1
  Sum of Elements1/1 -> Correlation/1, Find Peak/4(In2)
  Counter/1 -> Find Peak/1(In1)
  Threshold/1 -> Find Peak/2(threshold)
  Enable/1 -> Find Peak/3(In4)
  Find Peak/1(Out1) -> Peak Location/1
  Find Peak/2(Out2) -> Found ZC Seq/1

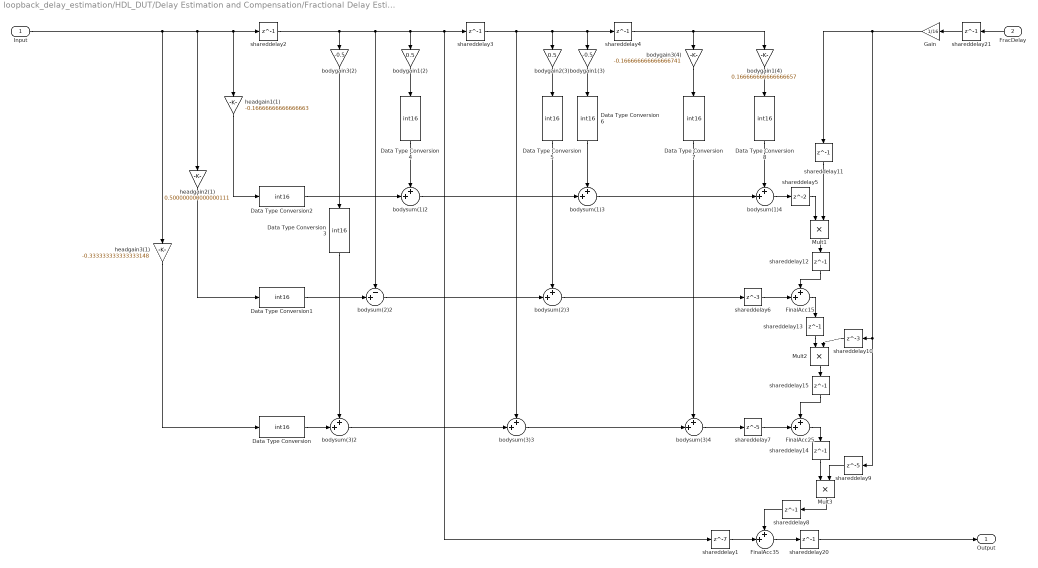
== system loopback_delay_estimation/HDL_DUT/Delay Estimation and Compensation/Fractional Delay Estimation/FarrowFractionalDelay ==
  Input : Inport
  FracDelay : Inport  Port=2
  Data Type Conversion{,1..8} (9 alike) : DataTypeConversion  OutDataTypeStr=int16
  FinalAcc15 : Sum  Inputs=++|  RndMeth=Nearest  SaturateOnIntegerOverflow=on  OutDataTypeStr=Inherit: Same as first input
  FinalAcc25 : Sum  Inputs=++|  RndMeth=Nearest  SaturateOnIntegerOverflow=on  OutDataTypeStr=Inherit: Same as first input
  FinalAcc35 : Sum  Inputs=++|  RndMeth=Nearest  SaturateOnIntegerOverflow=on
  Gain : Gain  Gain=1/16
  Mult1 : Product  RndMeth=Nearest  SaturateOnIntegerOverflow=on  OutDataTypeStr=Inherit: Same as first input
  Mult2 : Product  RndMeth=Nearest  SaturateOnIntegerOverflow=on  OutDataTypeStr=Inherit: Same as first input
  Mult3 : Product  RndMeth=Nearest  SaturateOnIntegerOverflow=on  OutDataTypeStr=Inherit: Same as first input
  bodygain1(2) : Gain  Gain=0.5  SaturateOnIntegerOverflow=on
  bodygain1(3) : Gain  Gain=-0.5  SaturateOnIntegerOverflow=on
  bodygain1(4) : Gain  Gain=0.166666666666666657  SaturateOnIntegerOverflow=on
  bodygain2(3) : Gain  Gain=0.5  SaturateOnIntegerOverflow=on
  bodygain3(2) : Gain  Gain=-0.5  SaturateOnIntegerOverflow=on
  bodygain3(4) : Gain  Gain=-0.166666666666666741  SaturateOnIntegerOverflow=on
  bodysum(1)2 : Sum  Inputs=++|  RndMeth=Nearest  SaturateOnIntegerOverflow=on  OutDataTypeStr=Inherit: Same as first input
  bodysum(1)3 : Sum  Inputs=++|  RndMeth=Nearest  SaturateOnIntegerOverflow=on  OutDataTypeStr=Inherit: Same as first input
  bodysum(1)4 : Sum  Inputs=++|  RndMeth=Nearest  SaturateOnIntegerOverflow=on  OutDataTypeStr=Inherit: Same as first input
  bodysum(2)2 : Sum  Inputs=-+|  RndMeth=Nearest  SaturateOnIntegerOverflow=on  OutDataTypeStr=Inherit: Same as first input
  bodysum(2)3 : Sum  Inputs=++|  RndMeth=Nearest  SaturateOnIntegerOverflow=on  OutDataTypeStr=Inherit: Same as first input
  bodysum(3)2 : Sum  Inputs=++|  RndMeth=Nearest  SaturateOnIntegerOverflow=on  OutDataTypeStr=Inherit: Same as first input
  bodysum(3)3 : Sum  Inputs=++|  RndMeth=Nearest  SaturateOnIntegerOverflow=on  OutDataTypeStr=Inherit: Same as first input
  bodysum(3)4 : Sum  Inputs=++|  RndMeth=Nearest  SaturateOnIntegerOverflow=on  OutDataTypeStr=Inherit: Same as first input
  headgain1(1) : Gain  Gain=-0.16666666666666663  SaturateOnIntegerOverflow=on
  headgain2(1) : Gain  Gain=0.500000000000000111  SaturateOnIntegerOverflow=on
  headgain3(1) : Gain  Gain=-0.333333333333333148  SaturateOnIntegerOverflow=on
  shareddelay1 : Delay  DelayLength=7  InitialCondition=0  InputProcessing=Columns as channels (frame based)
  shareddelay10 : Delay  DelayLength=3  InitialCondition=0  InputProcessing=Columns as channels (frame based)
  shareddelay{2..4,8,11..15,20..21} (11 alike) : Delay  DelayLength=1  InitialCondition=0  InputProcessing=Columns as channels (frame based)
  shareddelay5 : Delay  InitialCondition=0  InputProcessing=Columns as channels (frame based)
  shareddelay6 : Delay  DelayLength=3  InitialCondition=0  InputProcessing=Columns as channels (frame based)
  shareddelay7 : Delay  DelayLength=5  InitialCondition=0  InputProcessing=Columns as channels (frame based)
  shareddelay9 : Delay  DelayLength=5  InitialCondition=0  InputProcessing=Columns as channels (frame based)
  Output : Outport  VectorParamsAs1DForOutWhenUnconnected=off
  wires:
  bodysum(1)2/1 -> bodysum(1)3/2
  bodysum(2)2/1 -> bodysum(2)3/2
  bodysum(3)2/1 -> bodysum(3)3/2
  bodysum(1)3/1 -> bodysum(1)4/2
  bodysum(2)3/1 -> shareddelay6/1
  bodysum(3)3/1 -> bodysum(3)4/2
  bodygain3(4)/1 -> Data Type Conversion7/1
  bodysum(1)4/1 -> shareddelay5/1
  bodysum(3)4/1 -> shareddelay7/1
  shareddelay4/1 -> bodygain1(4)/1, bodygain3(4)/1
  FracDelay/1 -> shareddelay21/1
  Mult1/1 -> shareddelay12/1
  FinalAcc15/1 -> shareddelay13/1
  Mult2/1 -> shareddelay15/1
  FinalAcc25/1 -> shareddelay14/1
  Mult3/1 -> shareddelay8/1
  shareddelay20/1 -> Output/1
  FinalAcc35/1 -> shareddelay20/1
  Gain/1 -> shareddelay9/1, shareddelay10/1, shareddelay11/1
  Input/1 -> headgain1(1)/1, shareddelay2/1, headgain2(1)/1, headgain3(1)/1
  shareddelay1/1 -> FinalAcc35/2
  shareddelay7/1 -> FinalAcc25/2
  shareddelay6/1 -> FinalAcc15/2
  shareddelay5/1 -> Mult1/1
  headgain3(1)/1 -> Data Type Conversion/1
  bodygain3(2)/1 -> Data Type Conversion3/1
  shareddelay3/1 -> bodysum(3)3/1, bodygain1(3)/1, shareddelay4/1, bodygain2(3)/1
  Data Type Conversion7/1 -> bodysum(3)4/1
  headgain2(1)/1 -> Data Type Conversion1/1
  shareddelay2/1 -> shareddelay3/1, shareddelay1/1, bodygain1(2)/1, bodysum(2)2/1, bodygain3(2)/1
  bodygain2(3)/1 -> Data Type Conversion5/1
  headgain1(1)/1 -> Data Type Conversion2/1
  bodygain1(2)/1 -> Data Type Conversion4/1
  bodygain1(4)/1 -> Data Type Conversion8/1
  bodygain1(3)/1 -> Data Type Conversion6/1
  Data Type Conversion/1 -> bodysum(3)2/2
  Data Type Conversion1/1 -> bodysum(2)2/2
  Data Type Conversion2/1 -> bodysum(1)2/2
  Data Type Conversion3/1 -> bodysum(3)2/1
  Data Type Conversion4/1 -> bodysum(1)2/1
  Data Type Conversion5/1 -> bodysum(2)3/1
  Data Type Conversion6/1 -> bodysum(1)3/1
  Data Type Conversion8/1 -> bodysum(1)4/1
  shareddelay21/1 -> Gain/1
  shareddelay8/1 -> FinalAcc35/1
  shareddelay9/1 -> Mult3/2
  shareddelay10/1 -> Mult2/2
  shareddelay11/1 -> Mult1/2
  shareddelay12/1 -> FinalAcc15/1
  shareddelay13/1 -> Mult2/1
  shareddelay14/1 -> Mult3/1
  shareddelay15/1 -> FinalAcc25/1

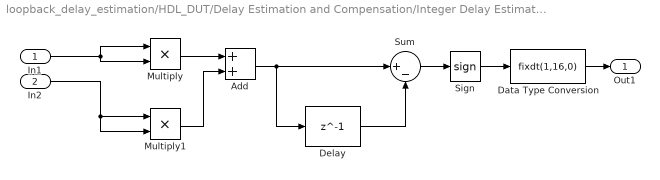
== system loopback_delay_estimation/HDL_DUT/Delay Estimation and Compensation/Integer Delay Estimation/Amplitude-Difference ==
  In1 : Inport
  In2 : Inport  Port=2
  Add : Sum
  Data Type Conversion : DataTypeConversion  OutDataTypeStr=fixdt(1,16,0)  SaturateOnIntegerOverflow=on
  Delay : Delay  DelayLength=1  InitialCondition=0  UseCircularBuffer=on
  Multiply : Product  OutDataTypeStr=int32
  Multiply1 : Product  OutDataTypeStr=int32
  Sign : Signum
  Sum : Sum  Inputs=|+-
  Out1 : Outport  VectorParamsAs1DForOutWhenUnconnected=off
  wires:
  Sum/1 -> Sign/1
  Add/1 -> Delay/1, Sum/1
  Multiply/1 -> Add/1
  Multiply1/1 -> Add/2
  Delay/1 -> Sum/2
  Sign/1 -> Data Type Conversion/1
  Data Type Conversion/1 -> Out1/1
  In1/1 -> Multiply/2, Multiply/1
  In2/1 -> Multiply1/2, Multiply1/1

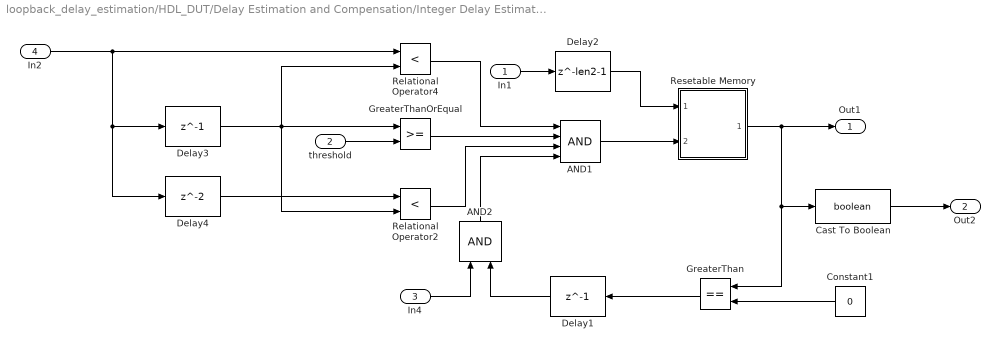
== system loopback_delay_estimation/HDL_DUT/Delay Estimation and Compensation/Integer Delay Estimation/Find Peak ==
  In1 : Inport
  threshold : Inport  Port=2
  In4 : Inport  Port=3
  In2 : Inport  Port=4
  AND1 : Logic  Inputs=4  AllPortsSameDT=off  OutDataTypeStr=boolean
  AND2 : Logic  AllPortsSameDT=off  OutDataTypeStr=boolean
  Cast To Boolean : DataTypeConversion  OutDataTypeStr=boolean
  Constant1 : Constant  Value=0  OutDataTypeStr=uint16  SampleTime=-1
  Delay1 : Delay  DelayLength=1  InitialCondition=0  UseCircularBuffer=on
  Delay2 : Delay  DelayLength=len2-1  InitialCondition=0  UseCircularBuffer=on
  Delay3 : Delay  DelayLength=1  InitialCondition=0  UseCircularBuffer=on
  Delay4 : Delay  InitialCondition=0  UseCircularBuffer=on
  GreaterThan : RelationalOperator  Operator===  OutDataTypeStr=boolean  RndMeth=Simplest
  GreaterThanOrEqual : RelationalOperator  OutDataTypeStr=boolean  RndMeth=Simplest
  Relational Operator2 : RelationalOperator  Operator=<  OutDataTypeStr=boolean  RndMeth=Nearest
  Relational Operator4 : RelationalOperator  Operator=<  OutDataTypeStr=boolean  RndMeth=Nearest
  Resetable Memory : Subsystem
  Out1 : Outport
  Out2 : Outport  Port=2
  wires:
  Delay1/1 -> AND2/2
  Delay3/1 -> GreaterThanOrEqual/1, Relational Operator4/2, Relational Operator2/2
  Relational Operator4/1 -> AND1/1
  Delay4/1 -> Relational Operator2/1
  AND2/1 -> AND1/4
  threshold/1 -> GreaterThanOrEqual/2
  GreaterThan/1 -> Delay1/1
  GreaterThanOrEqual/1 -> AND1/2
  Relational Operator2/1 -> AND1/3
  In1/1 -> Delay2/1
  In2/1 -> Relational Operator4/1, Delay4/1, Delay3/1
  In4/1 -> AND2/1
  Delay2/1 -> Resetable Memory/1(counter)
  AND1/1 -> Resetable Memory/2(trigger)
  Constant1/1 -> GreaterThan/2
  Resetable Memory/1(held counter) -> Out1/1, Cast To Boolean/1, GreaterThan/1
  Cast To Boolean/1 -> Out2/1

== system loopback_delay_estimation/HDL_DUT/Delay Estimation and Compensation/Integer Delay Estimation/Find Peak/Resetable Memory ==
  note: Reset when counter==0
  counter : Inport
  trigger : Inport  Port=2
  Compare To Zero : simulink/Logic and Bit Operations/Compare To Zero  relop=<=  OutDataTypeStr=boolean
  Constant1 : Constant  Value=0  OutDataTypeStr=Inherit: Inherit via back propagation  SampleTime=-1
  Delay : Delay  DelayLength=1  InitialCondition=0
  Switch : Switch  Criteria=u2 > Threshold
  Switch1 : Switch  Criteria=u2 > Threshold
  held counter : Outport  VectorParamsAs1DForOutWhenUnconnected=off
  wires:
  Switch/1 -> Switch1/3, held counter/1
  counter/1 -> Compare To Zero/1, Switch/1
  trigger/1 -> Switch/2
  Constant1/1 -> Switch1/1
  Compare To Zero/1 -> Switch1/2
  Delay/1 -> Switch/3
  Switch1/1 -> Delay/1
